simulink model "sim"  (R2023b)
settings: Solver=VariableStepAuto  StartTime=0.0  StopTime=10.0  RelTol=1e-3
libraries: aerolibadyn x1, aerolibatmos2 x1, simulink x1
settings Model: Creator=David  LastModifiedBy=David

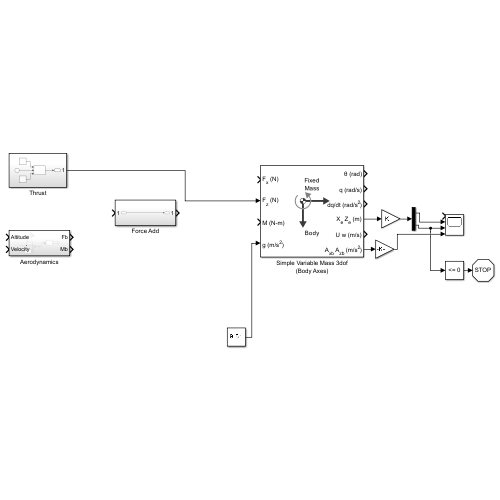
[thumbnail: Simulink's stored preview of the top-level diagram]
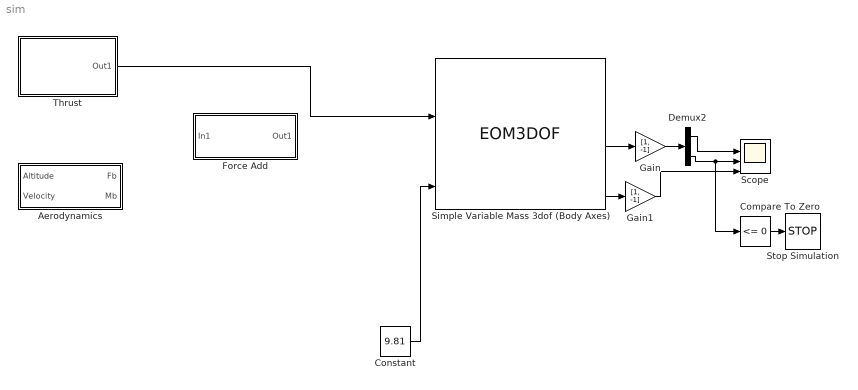
== system sim ==
  Aerodynamics : Subsystem
  Compare To Zero : simulink/Logic and Bit Operations/Compare To Zero  relop=<=  OutDataTypeStr=boolean
  Constant : Constant  Value=9.81
  Demux2 : Demux  Outputs=2
  Force Add : Subsystem
  Gain : Gain  Gain=[1, -1]
  Gain1 : Gain  Gain=[1, -1]
  Scope : Scope  NumInputPorts=4
  Simple Variable Mass 3dof (Body Axes) : EOM3DOF  v_ini=0  pos_ini=[0 -10]  mass=10  g_in=External
  Stop Simulation : Stop
  Thrust : Subsystem
  wires:
  Constant/1 -> Simple Variable Mass 3dof (Body Axes)/4
  Simple Variable Mass 3dof (Body Axes)/4 -> Gain/1
  Demux2/1 -> Scope/2
  Demux2/2 -> Compare To Zero/1, Scope/3
  Compare To Zero/1 -> Stop Simulation/1
  Gain/1 -> Demux2/1
  Simple Variable Mass 3dof (Body Axes)/6 -> Gain1/1
  Gain1/1 -> Scope/4
  Thrust/1(Out1) -> Simple Variable Mass 3dof (Body Axes)/2

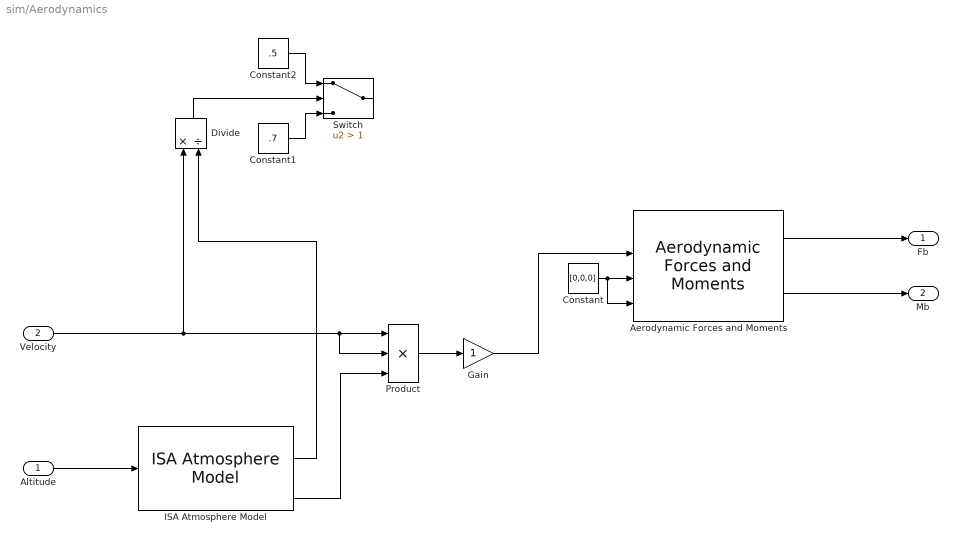
== system sim/Aerodynamics ==
  Altitude : Inport
  Velocity : Inport  Port=2
  "Aerodynamic Forces and Moments " : aerolibadyn/Aerodynamic Forces and Moments   inputAxes=Body  outputForceAxes=Body  outputMomentAxes=Body  S=1  b=1  cbar=1
  Constant : Constant  Value=[0,0,0]
  Constant1 : Constant  Value=.7
  Constant2 : Constant  Value=.5
  Divide : Product  Inputs=*/
  Gain : Gain
  ISA Atmosphere Model : aerolibatmos2/ISA Atmosphere Model  useExtended=off  action=Warning  custom=off  viscosityOut=off  g=9.80665  gamma=1.4  R=287.0531  L=0.0065  h_trop=11000  h_strat=20000  rho0=1.225  P0=101325  T0=288.15  h0=0
  Product : Product  Inputs=3
  Switch : Switch  Criteria=u2 > Threshold  Threshold=1  SaturateOnIntegerOverflow=off  InputSameDT=off
  Fb : Outport
  Mb : Outport  Port=2
  wires:
  "Aerodynamic Forces and Moments "/1 -> Fb/1
  "Aerodynamic Forces and Moments "/2 -> Mb/1
  Altitude/1 -> ISA Atmosphere Model/1
  ISA Atmosphere Model/4 -> Product/3
  Velocity/1 -> Divide/1, Product/2, Product/1
  Product/1 -> Gain/1
  Gain/1 -> "Aerodynamic Forces and Moments "/2
  ISA Atmosphere Model/2 -> Divide/2
  Constant/1 -> "Aerodynamic Forces and Moments "/4, "Aerodynamic Forces and Moments "/3
  Divide/1 -> Switch/2
  Constant1/1 -> Switch/3
  Constant2/1 -> Switch/1

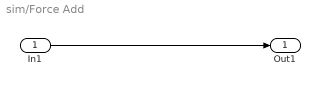
== system sim/Force Add ==
  In1 : Inport
  Out1 : Outport
  wires:
  In1/1 -> Out1/1

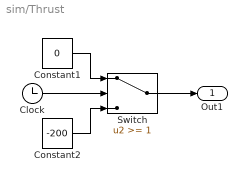
== system sim/Thrust ==
  Clock : Clock
  Constant1 : Constant  Value=0
  Constant2 : Constant  Value=-200
  Switch : Switch  Threshold=1  SaturateOnIntegerOverflow=off  InputSameDT=off
  Out1 : Outport
  wires:
  Constant2/1 -> Switch/3
  Clock/1 -> Switch/2
  Constant1/1 -> Switch/1
  Switch/1 -> Out1/1
